simulink model "testFrame_AngleCalculation"  (R2022b)
settings: Solver=FixedStepDiscrete  StartTime=0.0  StopTime=10  FixedStep=200e-6  RelTol=1e-3
libraries: simulink x5
settings Model: DataDictionary=PWMtoAngle.sldd  SnapshotInterval=1  Creator=unix  LastModifiedBy=unix
settings SolverCC: AlgebraicLoopSolver=TrustRegion
settings DebuggingCC: IntegerOverflowMsg=error  ParameterUnderflowMsg=error  UnconnectedInputMsg=warning  UnconnectedOutputMsg=warning  UnconnectedLineMsg=warning  SFMachineParentedDataDiag=warning  IntegerSaturationMsg=error
settings ModelReferenceCC: EnableRefExpFcnMdlSchedulingChecks=on
settings RTWCC: DLArmComputeVersion=19.05

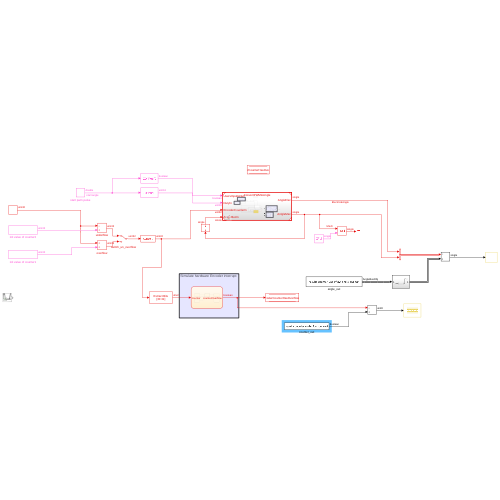
[thumbnail: Simulink's stored preview of the top-level diagram]
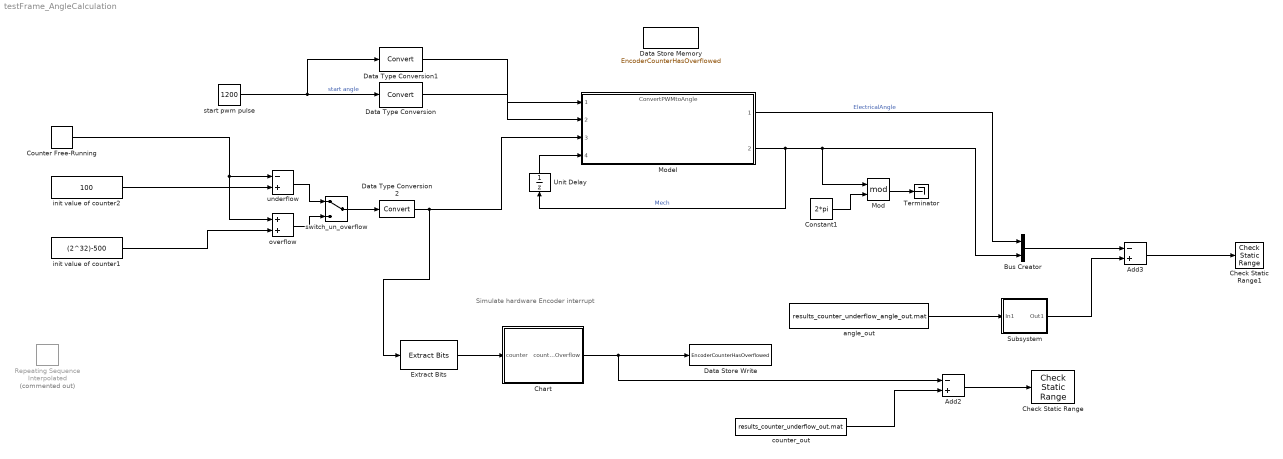
== system testFrame_AngleCalculation ==
  note: Simulate hardware Encoder interrupt
  Add2 : Sum  Inputs=-+
  Add3 : Sum  Inputs=-+
  Bus Creator : BusCreator  Inputs=2  OutDataTypeStr=Bus: AngleBusObj
      settings: InheritFromInputs=off
  Chart : Stateflow chart  TreatAsAtomicUnit=on
  Check Static Range : simulink/Model Verification/Check  Static Range  Description=-0.1 <= u <= 0.1  max=0.1  max_included=on  min=-0.1  min_included=on  enabled=on  stopWhenAssertionFail=on  export=off  icon=graphic
  Check Static Range1 : simulink/Model Verification/Check  Static Range  Description=-0.1 <= u <= 0.1  max=0.1  max_included=on  min=-0.1  min_included=on  enabled=on  stopWhenAssertionFail=on  export=off  icon=graphic
  Constant1 : Constant  Value=2*pi  OutDataTypeStr=single
  Counter Free-Running : simulink/Sources/Counter Free-Running  NumBits=32  tsamp=-1
  Data Store Memory : DataStoreMemory  DataStoreName=EncoderCounterHasOverflowed  ReadBeforeWriteMsg=warning  WriteAfterWriteMsg=warning  WriteAfterReadMsg=warning  ShowAdditionalParam=off  StateMustResolveToSignalObject=on
  Data Store Write : DataStoreWrite  DataStoreName=EncoderCounterHasOverflowed  IndexOptions=Index vector (dialog)  Indices=1  OutputSizes=1
  Data Type Conversion : DataTypeConversion  SaturateOnIntegerOverflow=off  RndMeth=Floor
  Data Type Conversion1 : DataTypeConversion  SaturateOnIntegerOverflow=off  RndMeth=Floor
  Data Type Conversion2 : DataTypeConversion  SaturateOnIntegerOverflow=off  RndMeth=Floor
  Extract Bits : simulink/Logic and Bit Operations/Extract Bits  bitsToExtract=Range of bits  numBits=8  bitIdxRange=[30 31]  outScalingMode=Treat bit field as an integer
  Mod : Math  Operator=mod  OutputSignalType=real
  Model : ModelReference  ModelNameDialog=ConvertPWMtoAngle.slx  SimulationMode=Accelerator  ModelReferenceVersion=7.3
  Repeating Sequence Interpolated : simulink/Sources/Repeating Sequence Interpolated  Commented=on  OutValues=[254 255 0 1 2 1 0 255 254].'  TimeValues=[0 1*(1*2e-04) 2*(1*2e-04) 3*(1*2e-04) 4*(1*2e-04) 5*(1*2e-04) 6*(1*2e-04) 7*(1*2e-04) 8*(1*2e-04)].'  LookUpMeth=Interpolation-Use End Values  tsamp=-1  OutMin=[]  OutMax=[]  OutDataTypeStr=uint8  OutputDataTypeScalingMode=uint8  OutDataType=fixdt(0,8)  OutScaling=2^-10
  Subsystem : Subsystem
  Terminator : Terminator
  Unit Delay : UnitDelay  SampleTime=-1  HasFrameUpgradeWarning=on
  angle_out : FromFile  FileName=results_counter_underflow_angle_out.mat  OutDataTypeStr=Bus: AngleBusObj
  counter_out : FromFile  FileName=results_counter_underflow_out.mat
  init value of counter1 : Constant  Value=(2^32)-500  OutDataTypeStr=uint32
  init value of counter2 : Constant  Value=100  OutDataTypeStr=uint32
  overflow : Sum  OutDataTypeStr=uint32
  start pwm pulse : Constant  Value=1200  OutMax=2^12-1
  switch_un_overflow : ManualSwitch
  underflow : Sum  Inputs=-+  OutDataTypeStr=uint32
  wires:
  start pwm pulse/1 -> Data Type Conversion1/1, Data Type Conversion/1  "start angle"
  Data Type Conversion/1 -> Model/2
  Model/1 -> Bus Creator/1  "ElectricalAngle"
  Data Type Conversion1/1 -> Model/1
  Unit Delay/1 -> Model/4
  Counter Free-Running/1 -> overflow/1, underflow/1
  Data Type Conversion2/1 -> Extract Bits/1, Model/3
  Model/2 -> Bus Creator/2, Mod/1, Unit Delay/1  "Mech"
  Constant1/1 -> Mod/2
  Chart/1(counterOverflow) -> Add2/1, Data Store Write/1
  Extract Bits/1 -> Chart/1(counter)
  underflow/1 -> switch_un_overflow/1
  overflow/1 -> switch_un_overflow/2
  init value of counter1/1 -> overflow/2
  switch_un_overflow/1 -> Data Type Conversion2/1
  init value of counter2/1 -> underflow/2
  Bus Creator/1 -> Add3/1
  counter_out/1 -> Add2/2
  Add2/1 -> Check Static Range/1
  Add3/1 -> Check Static Range1/1
  Mod/1 -> Terminator/1
  angle_out/1 -> Subsystem/1(In1)
  Subsystem/1(Out1) -> Add3/2

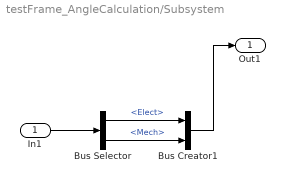
== system testFrame_AngleCalculation/Subsystem ==
  In1 : Inport
  Bus Creator1 : BusCreator  Inputs=2
  Bus Selector : BusSelector  OutputSignals=Elect,Mech
  Out1 : Outport
  wires:
  Bus Selector/2 -> Bus Creator1/2  "<Mech>"
  Bus Selector/1 -> Bus Creator1/1  "<Elect>"
  Bus Creator1/1 -> Out1/1
  In1/1 -> Bus Selector/1

== stateflow chart testFrame_AngleCalculation/Chart ==
  state pot_underflow
    en:counterOld=counter;
    du:counterOld=counter;
  state init_state
    en: counterOverflow=0;
  state pot_overflow
  state Counter_overflow1
    en: counterOverflow=1;
  state underflow
    en: counterOverflow=1;
  (default) -> init_state
  init_state -> pot_overflow [order 1] : [counter==3]
  init_state -> pot_underflow [order 2] : [counter==0]
  pot_underflow -> init_state [order 2] : [counter!=counterOld]
  pot_overflow -> Counter_overflow1 : [counter==0]
  pot_underflow -> underflow [order 1] : [counter==3]
  underflow -> init_state
  Counter_overflow1 -> init_state
  data: counter input; counterOverflow output; counterOld local uint32
